simulink model "sim_all"  (R2020a)
settings: Solver=VariableStepAuto  StartTime=0.0  StopTime=2000  RelTol=1e-3
values from neighbouring files (symbols this model uses):
  a1 = rho * D^4 * alpha1    (= 0.000388302366464)    [data_current.m]
  a2 = -rho * D^3 * alpha2 * (1 - omega)    (= 0.0037030698432)    [data_current.m]
  alpha1 = 0.0113    [data_current.m]
  alpha2 = -0.0091    [data_current.m]
  cornerA = [43.781381 ... (first row only)    [missionC.m]
  cornerB = [43.780975 ... (first row only)    [missionC.m]
  cornerC = [43.780189 ... (first row only)    [missionC.m]
  cornerD = [43.780602 ... (first row only)    [missionC.m]
  ctrl_clockwise = false    [controller.m]
  ctrl_int_bound_or = 0.1    [controller.m]
  ctrl_int_bound_pos = 1    [controller.m]
  ctrl_k_or = 1    [controller.m]
  ctrl_k_pos = 1/3    (= 0.333333333333)    [controller.m]
  ctrl_Ki_vel = 100    [controller.m]
  ctrl_Kp_v_pos = 200    [controller.m]
  ctrl_Kp_vel = 200    [controller.m]
  ctrl_TAM = [  1     1           0           0               0       0;               0     0           1           1               0       0;               0     0           0           0               1       1;               0     0  -(ctrl_r+ctrl_dc)  ctrl_r+ctrl_dc    0       0;               0     0           0           0            -ctrl_r    ctrl_r;           -ctrl_r ctrl_r        0           0       ...(+19 chars)    [controller.m]
  ctrl_Ts = 0.1    [controller.m]
  ctrl_va_uncontrolled = 0.15    [controller.m]
  ctrl_vel_uncontrolled = 0.5    [controller.m]
  D = 0.076    [data_current.m]
  dead_zone_limit = 31.5    [data_current.m]
  depth = 5    [missionC.m]
  distanceFromWall = 8    [missionC.m]
  initInspectedSide = 2    [missionC.m]
  initPoint = [ 43.780796 ... (first row only)    [missionC.m]
  mod_A = pi*mod_R*mod_R    [model.m]
  mod_Cd_F = 0.45    [model.m]
  mod_Cd_M = 0.4    [model.m]
  mod_eta_init = [mod_xNorth; mod_yEast; -mod_zDown; 0; 0; 0]    [model.m]
  mod_g = 9.81    [model.m]
  mod_h0 = 0    [model.m]
  mod_Ixx = mod_Io(1,1)    [model.m]
  mod_Iyy = mod_Io(2,2)    [model.m]
  mod_Izz = mod_Io(3,3)    [model.m]
  mod_Kp_dot = 0    [model.m]
  mod_lat0 = 43.780189    [model.m]
  mod_lon0 = 11.282698    [model.m]
  mod_m = 100    [model.m]
  mod_Mq_dot = mod_Kp_dot    (= 0)    [model.m]
  mod_ni_init = [0; 0; 0; 0; 0; 0]    [model.m]
  mod_Nr_dot = mod_Kp_dot    (= 0)    [model.m]
  mod_p1 = [0; mod_R; 0]    [model.m]
  mod_p2 = [0; -mod_R; 0]    [model.m]
  mod_p3 = [0; 0; (mod_R + mod_z_cm)]    [model.m]
  mod_p4 = [0; 0; -(mod_R + mod_z_cm)]    [model.m]
  mod_p5 = [mod_R; 0; 0]    [model.m]
  mod_p6 = [-mod_R; 0; 0]    [model.m]
  mod_R = ((3*mod_Vol)/(4*pi))^(1/3)    [model.m]
  mod_Rm = (4*mod_R)/(3*pi)    [model.m]
  mod_t1 = [1; 0; 0]    [model.m]
  mod_t2 = [1; 0; 0]    [model.m]
  mod_t3 = [0; 1; 0]    [model.m]
  mod_t4 = [0; 1; 0]    [model.m]
  mod_t5 = [0; 0; 1]    [model.m]
  mod_t6 = [0; 0; 1]    [model.m]
  mod_W = mod_m*mod_g    (= 981)    [model.m]
  mod_Xu_dot = (2/3)*mod_rho_AUV*pi*(mod_R^3)    [model.m]
  mod_Yv_dot = mod_Xu_dot    [model.m]
  mod_z_cm = mod_r_cm(3)    [model.m]
  mod_Zw_dot = mod_Xu_dot    [model.m]
  n_max = 340    [data_current.m]
  nav_DT = 0.1    [navigation.m]
  nav_filter = -1    [data_analysis_simulation_total.m]    (also in navigation.m)
  nav_giro = 2    [navigation.m]
  nav_h0 = 0    [navigation.m]
  nav_lat0 = cornerC(1)    [navigation.m]
  nav_lon0 = cornerC(2)    [navigation.m]
  nav_plane_AB = coefficient_plane(nav_A,nav_B)    [navigation.m]
  nav_plane_BC = coefficient_plane(nav_B,nav_C)    [navigation.m]
  nav_plane_CD = coefficient_plane(nav_C,nav_D)    [navigation.m]
  nav_plane_DA = coefficient_plane(nav_D,nav_A)    [navigation.m]
  nav_resampling = 10000    [navigation.m]
  omega = 0.1    [data_current.m]
  relativeDirection = 30    [missionC.m]
  res_enable_n_eff = 1    [navigation.m]
  rho = 1030    [data_current.m]
  sens_distCM = 0.267    [sensors.m]
  sens_Sample_time_AHRS = 0.1    [sensors.m]
  sens_Sample_time_depth = 0.1    [sensors.m]
  sens_Sample_time_dvl = 0.2    [sensors.m]
  sens_Sample_time_GPS = 1    [sensors.m]
  sens_Sample_time_GYRO = 0.1    [sensors.m]
  sens_Sample_time_sonar = 0.5    [sensors.m]
  sens_threshold = 0.485    [sensors.m]
  sens_Variance_AHRS_pitch = (0.0087)^2    (= 7.569e-05)    [sensors.m]
  sens_Variance_AHRS_roll = (0.0087)^2    (= 7.569e-05)    [sensors.m]
  sens_Variance_AHRS_yaw = (0.0017)^2    (= 2.89e-06)    [sensors.m]
  sens_Variance_depth1 = (0.2)^2    (= 0.04)    [sensors.m]
  sens_Variance_depth2 = (0.4)^2    (= 0.16)    [sensors.m]
  sens_Variance_DVL = (speed*0.03)^2    [sensors.m]
  sens_Variance_GPS = 3    [sensors.m]
  sens_Variance_GYRO = 2.5133e-06    [sensors.m]
  sens_Variance_sonar = 0.05    [sensors.m]
  soglia_or = [0.1, 0.1, 0.1]    [mission.m]
  soglia_orp = 0.1    [mission.m]
  soglia_parete = 0.5    [mission.m]
  soglia_parete_frenata = 0.5    [mission.m]
  soglia_pos = [0.00001, 0.00001, 0.5]    [mission.m]
  soglia_SOS_collisione = 2    [mission.m]
  soglia_SOS_or = [0.25, 0.25, 0.25]    [mission.m]
  soglia_SOS_orp = 0.25    [mission.m]
  soglia_SOS_parete = 1    [mission.m]
  soglia_SOS_pos = [0.00005, 0.00005, 1]    [mission.m]
  soglia_SOS_pos_ris = 2    [mission.m]
  soglia_SOS_vel = 0.2    [mission.m]
  SOS = 0    [mission.m]
  speed = 0.4    [missionC.m]
  stato = 100    [mission.m]
  timer = 40*2    (= 80)    [mission.m]
  Ts_supervisor = 0.1    [mission.m]
undefined symbols (not defined in the file or in its folder): DiscIntNeverNeededParam, nav_A, nav_B, nav_C, nav_D
libraries: simulink x8, cstblocks x6, simulink_extras x1
(part 8 of 8)

== matlab function sim_all/PF/SOS_flag_generator/MATLAB Function ==
  data: P_es input; SOS output; DVL input; AHRS input; gyro input; contatore input size=3 1; contatore output
%% Generazione flag di emergenza
% 1. Assenza di segnali dai sensori per un determinato tempo

function [SOS, contatore] = SOS_flag(P_es, DVL, AHRS, gyro, contatore)
    SOS=0;
 
    soglia_P = 10; %[m^2]
    if P_es(1,1)+P_es(2,2) > soglia_P || P_es(3,3) > soglia_P
        SOS=1;
    end
    
    if DVL == 1 
        contatore(1) = contatore(1) + 1;
    else
        contatore(1) = 0;
    end
    
    if AHRS == 1 
        contatore(2) = contatore(2) + 1;
    else
        contatore(2) = 0;
    end
    
    if gyro == 1 
        contatore(3) = contatore(3) + 1;
    else
        contatore(3) = 0;
    end
    
    if max(contatore) > 20
        SOS=1;
    end
    
    

end

== matlab function sim_all/Model/Vehicle Model/Acceleration Computation ==
  data: inertialTerm input; ni_dot output; mod_m parameter; mod_Ixx parameter; mod_Iyy parameter; mod_Izz parameter; mod_Xu_dot parameter; mod_Yv_dot parameter; mod_Zw_dot parameter; mod_Kp_dot parameter; mod_Mq_dot parameter; mod_Nr_dot parameter
function ni_dot = fcn(inertialTerm, mod_m, mod_Ixx, mod_Iyy, mod_Izz, mod_Xu_dot, mod_Yv_dot, mod_Zw_dot, mod_Kp_dot, mod_Mq_dot, mod_Nr_dot)

% Si definisce la matrice di inerzia del corpo rigido:
Mrb = [ mod_m   0   0   0   0   0;
        0   mod_m   0   0   0   0;
        0   0   mod_m   0   0   0;
        0   0   0  mod_Ixx  0   0;
        0   0   0   0  mod_Iyy  0;
        0   0   0   0   0  mod_Izz ];

% Si definisce la matrice di inerzia dovuta ai termini di massa e inerzia
% aggiunti:
Ma = [ -mod_Xu_dot     0        0        0        0        0;
          0     -mod_Yv_dot     0        0        0        0;
          0        0     -mod_Zw_dot     0        0        0;
          0        0        0     -mod_Kp_dot     0        0;
          0        0        0        0     -mod_Mq_dot     0;
          0        0        0        0        0     -mod_Nr_dot ];

M = Mrb + Ma;

ni_dot = M\inertialTerm;

== matlab function sim_all/Model/Vehicle Model/Coriolis term ==
  data: ni_rel input; mod_m parameter; mod_Ixx parameter; mod_Iyy parameter; mod_Izz parameter; mod_Xu_dot parameter; mod_Yv_dot parameter; mod_Zw_dot parameter; mod_Kp_dot parameter; Cterm output; mod_Mq_dot parameter; mod_Nr_dot parameter
function Cterm  = fcn(ni_rel, mod_m, mod_Ixx, mod_Iyy, mod_Izz, mod_Xu_dot, mod_Yv_dot, mod_Zw_dot, mod_Kp_dot, mod_Mq_dot, mod_Nr_dot)

u_rel = ni_rel(1);
v_rel = ni_rel(2);
w_rel = ni_rel(3);
p_rel = ni_rel(4);
q_rel = ni_rel(5);
r_rel = ni_rel(6);

% Si definisce la matrice di Coriolis del corpo rigido:
Crb = [    0          0          0           0          mod_m*w_rel     -mod_m*v_rel;
           0          0          0       -mod_m*w_rel          0         mod_m*u_rel;
           0          0          0        mod_m*v_rel      -mod_m*u_rel         0;
           0       mod_m*w_rel   -mod_m*v_rel        0        mod_Izz*r_rel   -mod_Iyy*q_rel;
       -mod_m*w_rel       0       mod_m*u_rel   -mod_Izz*r_rel         0       mod_Ixx*p_rel;
        mod_m*v_rel   -mod_m*u_rel       0       mod_Iyy*q_rel   -mod_Ixx*p_rel         0    ];

% Si definiscono i termini di Coriolis dovuti alle masse a alle inerzie
% aggiunte:
Ca = [      0              0              0              0        -mod_Zw_dot*w_rel   mod_Yv_dot*v_rel;
            0              0              0         mod_Zw_dot*w_rel        0        -mod_Xu_dot*u_rel;
            0              0              0        -mod_Yv_dot*v_rel   mod_Xu_dot*u_rel        0;
            0        -mod_Zw_dot*w_rel   mod_Yv_dot*v_rel        0        -mod_Nr_dot*r_rel   mod_Mq_dot*q_rel;
       mod_Zw_dot*w_rel        0        -mod_Xu_dot*u_rel   mod_Nr_dot*r_rel        0        -mod_Kp_dot*p_rel;
      -mod_Yv_dot*v_rel   mod_Xu_dot*u_rel        0        -mod_Mq_dot*q_rel   mod_Kp_dot*p_rel        0       ];

C = Crb + Ca;

Cterm = C*ni_rel;

== matlab function sim_all/Mission_supervisor_v3/Mission_Supervisor/Inizio/MATLAB Function ==
  data: current_state output; parete_attuale output; stato_interno output; Pos_d output size=3; Pos_s input; error_flag input; attesa input; initInspectedSide parameter; initPoint parameter; timer parameter; SOS parameter
function [current_state, parete_attuale, stato_interno, Pos_d] =  Inizio(Pos_s, error_flag, attesa, initInspectedSide, initPoint, timer, SOS)
    
    disp("Inizio");
    
    %% Unita' di misura
    
    % Pos_d, Pos_s, initPoint                                                [deg, deg, m]
    % attesa, timer                                                          [s]
    
    %% Inizializzazione variabili
    
    % Mantenimento di stato_interno al valore
    % desiderato durante la permanenza del sistema nello stato corrente.
    stato_interno = 100;

    % Se non si ricevono dati dal GPS per un tempo superiore ad una soglia
    % massima di attesa, la missione viene interrotta poiché non è
    % possibile localizzarsi nel bacino
    if ((isnan(Pos_s(1)) || isnan(Pos_s(2))) && (attesa > timer))
        SOS = 1;
        disp("EMERGENZA: mancata ricezione dati da GPS");
    end
    
    %% Preparazione dei riferimenti 
    
        % Parete di inizio pattugliamento
        parete_attuale = initInspectedSide;
        
        % Posizione di inizio missione
        Pos_d = initPoint; 
        
        
    %% Transizione di stato effettiva
    
        % Quando i riferimenti sono correttamente settati
        % viene comunicato agli altri moduli il passaggio di stato
        current_state = 100;  
        
    %% Decisione dello stato successivo
    
     if error_flag == 1
        disp("EMERGENZA: errore segnalato dagli altri sottosistemi");
        SOS = 1;
     end
    
    % Si verifica lo stato di emergenza e la ricezione di misure dal GPS
    if (SOS == 0 && ((isnan(Pos_s(1)) == false && isnan(Pos_s(2)) == false))) 
        
        stato_interno = 101;   % Si passa allo stato successivo
    else
        if SOS == 1
           
            stato_interno = 304; % Politica di emergenza: si passa in fine missione   
        end
    end

end

== matlab function sim_all/Model/Vehicle Model/Damping term ==
  data: ni_rel input; Dterm output; rho parameter; mod_Rm parameter; mod_A parameter; mod_Cd_F parameter; mod_Cd_M parameter
function Dterm = fcn(ni_rel, rho, mod_Rm, mod_A, mod_Cd_F, mod_Cd_M)

u_rel = ni_rel(1);
v_rel = ni_rel(2);
w_rel = ni_rel(3);
p_rel = ni_rel(4);
q_rel = ni_rel(5);
r_rel = ni_rel(6);

%Termine costante di Damping rispettivamente riferito alle forze e ai momenti
Dconst_F = 0.5*rho*mod_Cd_F*mod_A;
Dconst_M = 0.5*rho*mod_Cd_M*mod_A*mod_Rm*mod_Rm*mod_Rm;

% Si definiscono i termini diagonali della matrice di Damping:
D1 = Dconst_F*abs(u_rel)*u_rel;
D2 = Dconst_F*abs(v_rel)*v_rel;
D3 = Dconst_F*abs(w_rel)*w_rel;
D4 = Dconst_M*abs(p_rel)*p_rel;
D5 = Dconst_M*abs(q_rel)*q_rel; 
D6 = Dconst_M*abs(r_rel)*r_rel; 

Dterm = [D1; D2; D3; D4; D5; D6];

== matlab function sim_all/Model/Vehicle Model/Gravitational terms ==
  data: eta input; Gterm output; mod_W parameter; mod_z_cm parameter; mod_R parameter; rho parameter; mod_g parameter
function Gterm = fcn (eta, mod_W, mod_z_cm, mod_R, rho, mod_g)

% Si definisce il vettore delle forze e dei momenti gravitazionali 
% considerando una forza di galleggiamento variabile al variare del volume 
% del veicolo immerso.

z = eta(3);
phi = eta(4);
theta = eta(5);
 
% Si definisce la componente z del vettore posizione del centro di
% galleggiamento rispetto al centro di massa:
z_CB = -0.1;

% Caso di veicolo totalmente immerso:
if (z >= mod_R + mod_z_cm)
    G = [0; 0; 0; mod_z_cm*mod_W*cos(theta)*sin(phi); mod_z_cm*mod_W*sin(theta); 0];

% Caso di veicolo parzialmente immerso (forza di galleggiamento variabile):
elseif (z >= -(mod_R - mod_z_cm) && z < (mod_R + mod_z_cm))
    Vol_immerso = pi*((z+mod_R-mod_z_cm)^2)*(mod_R-((z+mod_R-mod_z_cm)/3));
    B = rho*mod_g*Vol_immerso;
    G = [(mod_W-B)*sin(theta); -(mod_W-B)*cos(theta)*sin(phi); -(mod_W-B)*cos(theta)*cos(phi); -z_CB*B*cos(theta)*sin(phi); -z_CB*B*sin(theta); 0];

% Caso di veicolo completamente emerso (condizione che non si deve verificare per nessun motivo):
else
    G = [mod_W*sin(theta); -mod_W*cos(theta)*sin(phi); -mod_W*cos(theta)*cos(phi); 0; 0; 0];    
end

Gterm = G;

== matlab function sim_all/Model/Vehicle Model/Kinematic Model ==
  data: eta input; ni input; eta_dot output
function eta_dot = fcn(eta, ni)

phi = eta(4);
theta = eta(5); 
psi = eta(6);

% Si definisce la matrice di rotazione J1 che mappa la velocità lineare in 
% terna body nella velocità lineare in terna NED: 
J1 = [ cos(psi)*cos(theta)   -sin(psi)*cos(phi) + (cos(psi)*sin(theta)*sin(phi))   (sin(psi)*sin(phi)) + (cos(psi)*cos(phi)*sin(theta));
       sin(psi)*cos(theta)   (cos(psi)*cos(phi)) + (sin(psi)*sin(theta)*sin(phi))  (-cos(psi)*sin(phi)) + (sin(psi)*sin(theta)*cos(phi));
      -sin(theta)             cos(theta)*sin(phi)                                   cos(theta)*cos(phi)                                  ];

% Si definisce la matrice J2 che mappa la velocità angolare in terna body
% nel vettore orientazione espresso in terna NED (J2 non è una matrice di 
% rotazione):
J2 = [ 1   sin(phi)*tan(theta)   cos(phi)*tan(theta);
       0   cos(phi)             -sin(phi);
       0   sin(phi)/cos(theta)   cos(phi)/cos(theta) ];
       
J = [   J1      zeros(3);
      zeros(3)    J2     ];

eta_dot = J*ni;

== matlab function sim_all/Model/Vehicle Model/P1/Propeller1 ==
  data: n1 input; T1 output; V1 input; D parameter; omega parameter; a1 parameter; a2 parameter; alpha1 parameter; alpha2 parameter
function T1 = thrusterModel(n1, V1, D, omega, a1, a2, alpha1, alpha2)

Va1 = (1-omega) * V1;     % Advancement velocity at the propeller
J0 = Va1/(n1*D);          % Advancement Coefficient

if J0 > -alpha1/alpha2  % Out of linearity domain (right side)
    T1 = 0;              % A null generated thrust is assumed
    
elseif J0 < 0           % Out of linearity domain (left side)
    T1 = a1*abs(n1)*n1;    % Bollard thrust is assumed

else                    % Within the linearity domain
    T1 = a1*abs(n1)*n1 - a2*abs(n1)*V1;
end

== matlab function sim_all/Model/Vehicle Model/P2/Propeller2 ==
  data: n2 input; T2 output; V2 input; D parameter; omega parameter; a1 parameter; a2 parameter; alpha1 parameter; alpha2 parameter
function T2 = thrusterModel(n2, V2, D, omega, a1, a2, alpha1, alpha2)

Va2 = (1-omega) * V2;     % Advancement velocity at the propeller
J0 = Va2/(n2*D);          % Advancement Coefficient

if J0 > -alpha1/alpha2  % Out of linearity domain (right side)
    T2 = 0;              % A null generated thrust is assumed
    
elseif J0 < 0           % Out of linearity domain (left side)
    T2 = a1*abs(n2)*n2;    % Bollard thrust is assumed

else                    % Within the linearity domain
    T2 = a1*abs(n2)*n2 - a2*abs(n2)*V2;
end

== matlab function sim_all/Model/Vehicle Model/P3/Propeller3 ==
  data: n3 input; T3 output; V3 input; D parameter; omega parameter; a1 parameter; a2 parameter; alpha1 parameter; alpha2 parameter
function T3 = thrusterModel(n3, V3, D, omega, a1, a2, alpha1, alpha2)

Va3 = (1-omega) * V3;     % Advancement velocity at the propeller
J0 = Va3/(n3*D);          % Advancement Coefficient

if J0 > -alpha1/alpha2  % Out of linearity domain (right side)
    T3 = 0;              % A null generated thrust is assumed
    
elseif J0 < 0           % Out of linearity domain (left side)
    T3 = a1*abs(n3)*n3;    % Bollard thrust is assumed

else                    % Within the linearity domain
    T3 = a1*abs(n3)*n3 - a2*abs(n3)*V3;
end

== matlab function sim_all/Model/Vehicle Model/P4/Propeller4 ==
  data: n4 input; T4 output; V4 input; D parameter; omega parameter; a1 parameter; a2 parameter; alpha1 parameter; alpha2 parameter
function T4 = thrusterModel(n4, V4, D, omega, a1, a2, alpha1, alpha2)

Va4 = (1-omega) * V4;     % Advancement velocity at the propeller
J0 = Va4/(n4*D);          % Advancement Coefficient

if J0 > -alpha1/alpha2  % Out of linearity domain (right side)
    T4 = 0;              % A null generated thrust is assumed
    
elseif J0 < 0           % Out of linearity domain (left side)
    T4 = a1*abs(n4)*n4;    % Bollard thrust is assumed

else                    % Within the linearity domain
    T4 = a1*abs(n4)*n4 - a2*abs(n4)*V4;
end

== matlab function sim_all/Model/Vehicle Model/P5/Propeller5 ==
  data: n5 input; T5 output; V5 input; D parameter; omega parameter; a1 parameter; a2 parameter; alpha1 parameter; alpha2 parameter
function T5 = thrusterModel(n5, V5, D, omega, a1, a2, alpha1, alpha2)

Va5 = (1-omega) * V5;     % Advancement velocity at the propeller
J0 = Va5/(n5*D);          % Advancement Coefficient

if J0 > -alpha1/alpha2  % Out of linearity domain (right side)
    T5 = 0;              % A null generated thrust is assumed
    
elseif J0 < 0           % Out of linearity domain (left side)
    T5 = a1*abs(n5)*n5;    % Bollard thrust is assumed

else                    % Within the linearity domain
    T5 = a1*abs(n5)*n5 - a2*abs(n5)*V5;
end

== matlab function sim_all/Model/Vehicle Model/P6/Propeller6 ==
  data: n6 input; T6 output; V6 input; D parameter; omega parameter; a1 parameter; a2 parameter; alpha1 parameter; alpha2 parameter
function T6 = thrusterModel(n6, V6, D, omega, a1, a2, alpha1, alpha2)

Va6 = (1-omega) * V6;     % Advancement velocity at the propeller
J0 = Va6/(n6*D);          % Advancement Coefficient

if J0 > -alpha1/alpha2  % Out of linearity domain (right side)
    T6 = 0;              % A null generated thrust is assumed
    
elseif J0 < 0           % Out of linearity domain (left side)
    T6 = a1*abs(n6)*n6;    % Bollard thrust is assumed

else                    % Within the linearity domain
    T6 = a1*abs(n6)*n6 - a2*abs(n6)*V6;
end

== matlab function sim_all/Model/Vehicle Model/TAM ==
  data: T1 input; tau output; T2 input; T3 input; T4 input; T5 input; T6 input; eta input; mod_R parameter; mod_z_cm parameter
function tau = fcn (T1, T2, T3, T4, T5, T6, eta, mod_R, mod_z_cm)

% Si definisce il vettore delle forze e dei momenti applicati al veicolo al 
% variare dei propulsori immersi o emersi, si assume che i propulsori non 
% funzionino se utilizzati fuori dall'acqua. Si assume inoltre che il
% veicolo esca fuori dall'acqua orizzontalmente (con angoli di pitch e roll
% nulli).

z = eta(3);

% Veicolo completamente immerso, tutti i propulsori funzionano.
if (z >= (mod_R+mod_z_cm)) 
    tau1 = T1 + T2;
    tau2 = T3 + T4;
    tau3 = T5 + T6;
    tau4 = ((-(mod_R+mod_z_cm))*T3) + ((mod_R+mod_z_cm)*T4);
    tau5 = (-mod_R*T5) + (mod_R*T6);
    tau6 = (-mod_R*T1) + (mod_R*T2);
    
% Veicolo emerso in un range che va al dall'estremo superiore fino al 
% centro di massa (il centro di massa è ancora immerso), funzionano tutti i 
% propulsori tranne P4.
elseif (z >= 0 && z < (mod_R+mod_z_cm)) 
    tau1 = T1 + T2;
    tau2 = T3;
    tau3 = T5 + T6;
    tau4 = ((-(mod_R+mod_z_cm))*T3);
    tau5 = (-mod_R*T5) + (mod_R*T6);
    tau6 = (-mod_R*T1) + (mod_R*T2);

% Veicolo immerso in un range che va dall'estremo inferiore fino al centro 
% di massa (il centro di massa è emerso), funziona solo il propulsore P3.
elseif (z >= -(mod_R+mod_z_cm) && z < 0)
    tau1 = 0;
    tau2 = T3;
    tau3 = 0;
    tau4 = ((-(mod_R+mod_z_cm))*T3);
    tau5 = 0;
    tau6 = 0;

% Veicolo completamente emerso, nessun propulsore funziona.
else
    tau1 = 0;
    tau2 = 0;
    tau3 = 0;
    tau4 = 0;
    tau5 = 0;
    tau6 = 0;
end

tau = [tau1; tau2; tau3; tau4; tau5; tau6];

== matlab function sim_all/Model/Vehicle Model/Thruster Velocity Computation ==
  data: V1 output; V2 output; V3 output; V4 output; V5 output; V6 output; ni_rel input; mod_p1 parameter; mod_p2 parameter; mod_p3 parameter; mod_p4 parameter; mod_p5 parameter; mod_p6 parameter; mod_t1 parameter; mod_t2 parameter; mod_t3 parameter; mod_t4 parameter; mod_t5 parameter; mod_t6 parameter
function [V1, V2, V3, V4, V5, V6] = fcn(ni_rel, mod_p1, mod_p2, mod_p3, mod_p4, mod_p5, mod_p6, mod_t1, mod_t2, mod_t3, mod_t4, mod_t5, mod_t6)

% Si spezza il vettore velocità relativa nella componente lineare e angolare:
ni1_rel = [ni_rel(1); ni_rel(2); ni_rel(3)];
ni2_rel = [ni_rel(4); ni_rel(5); ni_rel(6)];

% Si definiscono i vettori velocità dei propulsori: 
Vp1 = ni1_rel + cross(ni2_rel, mod_p1);
Vp2 = ni1_rel + cross(ni2_rel, mod_p2);
Vp3 = ni1_rel + cross(ni2_rel, mod_p3);
Vp4 = ni1_rel + cross(ni2_rel, mod_p4);
Vp5 = ni1_rel + cross(ni2_rel, mod_p5);
Vp6 = ni1_rel + cross(ni2_rel, mod_p6);

% Si proiettano tali velocità lungo le direzioni date dai versori:
V1 = dot(Vp1, mod_t1); 
V2 = dot(Vp2, mod_t2);
V3 = dot(Vp3, mod_t3);
V4 = dot(Vp4, mod_t4);
V5 = dot(Vp5, mod_t5);
V6 = dot(Vp6, mod_t6);

== matlab function sim_all/Model/Vehicle Model/seaCurrent from NED to body ==
  data: seaCurrent_Velocity output; eta input; seaCurrent parameter
function seaCurrent_Velocity = fcn(eta, seaCurrent)

phi = eta(4);
theta = eta(5); 
psi = eta(6);

% Si definisce la matrice di rotazione J1 che mappa la velocità lineare 
% della corrente in terna body nella velocità lineare della corrente in 
% terna NED: 
J1 = [ cos(psi)*cos(theta)   -sin(psi)*cos(phi) + (cos(psi)*sin(theta)*sin(phi))   (sin(psi)*sin(phi)) + (cos(psi)*cos(phi)*sin(theta));
       sin(psi)*cos(theta)   (cos(psi)*cos(phi)) + (sin(psi)*sin(theta)*sin(phi))  (-cos(psi)*sin(phi)) + (sin(psi)*sin(theta)*cos(phi));
      -sin(theta)             cos(theta)*sin(phi)                                   cos(theta)*cos(phi)                                  ];

% Si definisce la matrice J1 inversa in maniera tale da mappare la velocità
% della corrente in terna NED nella velocità lineare della corrente in
% terna body (essendo J1 una matrice di rotazione l'inversa coincide con la
% trasposta):
J1_inv = J1';

%si definisce la velocità della corrente espressa in terna Body
seaCurrent_body = J1_inv*seaCurrent;
seaCurrent_Velocity = [seaCurrent_body; 0; 0; 0];

== matlab function sim_all/Mission_supervisor_v3/Mission_Supervisor/MATLAB Function ==
  data: parete_iniziale input; verso input; parete output; contatore input; initInspectedSide parameter; current_state input; giro output
function [parete, giro] = aggiorna_parete(parete_iniziale, verso, contatore, initInspectedSide,current_state)
   
 %% Corpo funzione 
    
    % A seconda del senso di pattugliamento si ha l'aggiornamento del valore
    % di parete attuale. 
    
    if(strcmp(verso,'clockwise') == 1)
        giro = 0;
        parete = mod((parete_iniziale + contatore),4);
        if(parete == 0)
            parete = 4;
        end
    else % 'counterclockwise'
        giro = 1;
        parete = parete_iniziale - contatore;
        if(parete <= 0)
            parete = parete+4;
        end
    end

    % Per stati precedenti al 201, si forza questa variabile a
    % mantenere il valore pari al valore iniziale. 
    if(current_state < 201)
        parete = initInspectedSide;
    end
    
end

== matlab function sim_all/Model/from NED to ECEF ==
  data: eta1 input; eta1_ECEF output; mod_lat0 parameter; mod_lon0 parameter; mod_h0 parameter
function eta1_ECEF = fcn(eta1, mod_lat0, mod_lon0, mod_h0)

eta1_ECEF = [0; 0; 0];

eta1_North = eta1(1);
eta1_East = eta1(2);
eta1_Down = eta1(3);

coder.extrinsic('evalin','wgs84Ellipsoid','ned2geodetic')

[lat_ECEF, lon_ECEF, h_ECEF] = ned2geodetic(eta1_North, eta1_East, eta1_Down, mod_lat0, mod_lon0, mod_h0, wgs84Ellipsoid);

eta1_ECEF = [lat_ECEF; lon_ECEF; h_ECEF];

== matlab function sim_all/Sensors/BLOCCO GYRO1/Subsystem/GEOD to NED ==
  data: Bias_G output; t input
function Bias_G  = fcn(t)
ramp=t*(3.8785e-05);
Bias_G=ramp;

== matlab function sim_all/Controller_mk4_v3/C_pos/abs_integrator2/Body2Ned ==
  data: x_b input size=[3 1]; x_n output size=[3 1]; or input
%% Da BODY a NED per integrazione assoluta
function x_n = body2ned(x_b,or)
C=zeros(3,3);
C=Cx(or(1))'*Cy(or(2))'*Cz(or(3))';
x_n = C*x_b;
end

== matlab function sim_all/Controller_mk4_v3/C_pos/abs_integrator2/Ned2Body1 ==
  data: x_n input size=[3 1]; x_b output size=[3 1]; or input
%% Da NED a BODY
function x_b = ned2body(x_n,or)
C=zeros(3,3);
C=Cx(or(1))'*Cy(or(2))'*Cz(or(3))';
x_b = C'*x_n;
end

== matlab function sim_all/Controller_mk4_v3/C_pos/abs_integrator1/Body2Ned ==
  data: x_b input size=[3 1]; x_n output size=[3 1]; or input
%% Da BODY a NED
function x_n = body2ned(x_b,or)
C=zeros(3,3);
C=Cx(or(1))'*Cy(or(2))'*Cz(or(3))';
x_n = C*x_b;
end

== matlab function sim_all/Controller_mk4_v3/C_pos/abs_integrator1/Ned2Body1 ==
  data: x_n input size=[3 1]; x_b output size=[3 1]; or input
%% Da NED a BODY
function x_b = ned2body(x_n,or)
C=zeros(3,3);
C=Cx(or(1))'*Cy(or(2))'*Cz(or(3))';
x_b = C'*x_n;
end

== matlab function sim_all/Controller_mk4_v3/C_vel/abs_integrator/Body2Ned ==
  data: x_b input size=[3 1]; x_n output size=[3 1]; or input
%% Da BODY a NED
function x_n = body2ned(x_b,or)
C=zeros(3,3);
C=Cx(or(1))'*Cy(or(2))'*Cz(or(3))';
x_n = C*x_b;
end

== matlab function sim_all/Controller_mk4_v3/C_vel/abs_integrator/Ned2Body1 ==
  data: x_n input size=[3 1]; x_b output size=[3 1]; or input
%% Da NED a BODY
function x_b = ned2body(x_n,or)
C=zeros(3,3);
C=Cx(or(1))'*Cy(or(2))'*Cz(or(3))';
x_b = C'*x_n;
end
